simulink model "GTA_PCMFirmware"  (Simulink 7.8)
settings: Solver=FixedStepDiscrete  StartTime=0.0  StopTime=10.0  RelTol=1e-3
PreLoadFcn:
  | try, eval([bdroot '_setup']); catch, eval('model_setup', ''); end
InitFcn:
  | try, eval([bdroot '_setup']); catch, eval('model_setup', ''); end
undefined symbols (not defined in the file): fndFwd, fndNeut, fndRev, FWDlockout, GCM, keySwIgn2, motohawk_build_version, motohawk_trunc_name, motohawk_vardec_path, REVlockout
libraries: MotoHawk_lib x313, simulink x47, GTA_Library x13
(part 6 of 7)

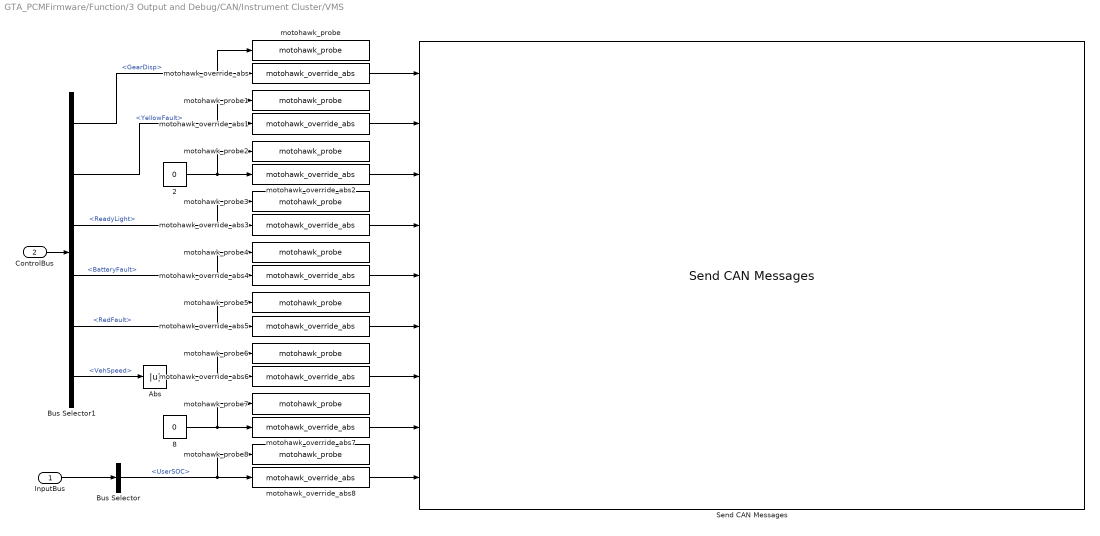
== system GTA_PCMFirmware/Function/3 Output and Debug/CAN/Instrument Cluster/VMS ==
  InputBus : Inport
  ControlBus : Inport  Port=2
  "   2" : Constant  Value=0  OutDataTypeStr=boolean
  "   8" : Constant  Value=0  OutDataTypeStr=uint8
  Abs : Abs
  Bus Selector : BusSelector  OutputSignals=CANin.BMS.csInfo.UserSOC
  Bus Selector1 : BusSelector  OutputSignals=Display.GearDisp,Display.FaultLamp.YellowFault,Display.ReadyLight,SYSin.BUS.Faults.BatteryFault.BatteryFault,Display.FaultLamp.RedFault,Display.VehSpeed
  Send CAN Messages : MotoHawk_lib/CAN Blocks/Send CAN Messages  bus=-2  nam='CAN_1'  msgl=CANMSG_ClusterVMS1  pace=5  labelwires=off
  motohawk_override_abs : MotoHawk_lib/Calibration & Probing Blocks/motohawk_override_abs  parent_name='GearboxDisplay'  parent_val=0  show_more=off  name_source=Use Parameter  parent_read_level=1  parent_override_level=1  view_as=Number  enum_struct={'Disabled', 'Enabled'}  use_help_units=off  parent_help=''  parent_units=''  use_min_max=off  parent_min=-inf  parent_max=inf  use_precision=off  parent_precision=''  parent_gain=1  parent_offset=0  parent_exp=1  use_mototune_group=off  parent_group=motohawk_vardec_path(gcb)
  motohawk_override_abs1 : MotoHawk_lib/Calibration & Probing Blocks/motohawk_override_abs  parent_name='YellowWarningLight'  parent_val=0  show_more=off  name_source=Use Parameter  parent_read_level=1  parent_override_level=1  view_as=Number  enum_struct={'Disabled', 'Enabled'}  use_help_units=off  parent_help=''  parent_units=''  use_min_max=off  parent_min=-inf  parent_max=inf  use_precision=off  parent_precision=''  parent_gain=1  parent_offset=0  parent_exp=1  use_mototune_group=off  parent_group=motohawk_vardec_path(gcb)
  motohawk_override_abs2 : MotoHawk_lib/Calibration & Probing Blocks/motohawk_override_abs  parent_name='SOCwarning'  parent_val=0  show_more=off  name_source=Use Parameter  parent_read_level=1  parent_override_level=1  view_as=Number  enum_struct={'Disabled', 'Enabled'}  use_help_units=off  parent_help=''  parent_units=''  use_min_max=off  parent_min=-inf  parent_max=inf  use_precision=off  parent_precision=''  parent_gain=1  parent_offset=0  parent_exp=1  use_mototune_group=off  parent_group=motohawk_vardec_path(gcb)
  motohawk_override_abs3 : MotoHawk_lib/Calibration & Probing Blocks/motohawk_override_abs  parent_name='ReadyLight'  parent_val=0  show_more=off  name_source=Use Parameter  parent_read_level=1  parent_override_level=1  view_as=Number  enum_struct={'Disabled', 'Enabled'}  use_help_units=off  parent_help=''  parent_units=''  use_min_max=off  parent_min=-inf  parent_max=inf  use_precision=off  parent_precision=''  parent_gain=1  parent_offset=0  parent_exp=1  use_mototune_group=off  parent_group=motohawk_vardec_path(gcb)
  motohawk_override_abs4 : MotoHawk_lib/Calibration & Probing Blocks/motohawk_override_abs  parent_name='BatteryWarning'  parent_val=0  show_more=off  name_source=Use Parameter  parent_read_level=1  parent_override_level=1  view_as=Number  enum_struct={'Disabled', 'Enabled'}  use_help_units=off  parent_help=''  parent_units=''  use_min_max=off  parent_min=-inf  parent_max=inf  use_precision=off  parent_precision=''  parent_gain=1  parent_offset=0  parent_exp=1  use_mototune_group=off  parent_group=motohawk_vardec_path(gcb)
  motohawk_override_abs5 : MotoHawk_lib/Calibration & Probing Blocks/motohawk_override_abs  parent_name='RedWarningLight'  parent_val=0  show_more=off  name_source=Use Parameter  parent_read_level=1  parent_override_level=1  view_as=Number  enum_struct={'Disabled', 'Enabled'}  use_help_units=off  parent_help=''  parent_units=''  use_min_max=off  parent_min=-inf  parent_max=inf  use_precision=off  parent_precision=''  parent_gain=1  parent_offset=0  parent_exp=1  use_mototune_group=off  parent_group=motohawk_vardec_path(gcb)
  motohawk_override_abs6 : MotoHawk_lib/Calibration & Probing Blocks/motohawk_override_abs  parent_name='VehicleSpeed'  parent_val=0  show_more=off  name_source=Use Parameter  parent_read_level=1  parent_override_level=1  view_as=Number  enum_struct={'Disabled', 'Enabled'}  use_help_units=off  parent_help=''  parent_units=''  use_min_max=off  parent_min=-inf  parent_max=inf  use_precision=off  parent_precision=''  parent_gain=1  parent_offset=0  parent_exp=1  use_mototune_group=off  parent_group=motohawk_vardec_path(gcb)
  motohawk_override_abs7 : MotoHawk_lib/Calibration & Probing Blocks/motohawk_override_abs  parent_name='Odometer'  parent_val=0  show_more=off  name_source=Use Parameter  parent_read_level=1  parent_override_level=1  view_as=Number  enum_struct={'Disabled', 'Enabled'}  use_help_units=off  parent_help=''  parent_units=''  use_min_max=off  parent_min=-inf  parent_max=inf  use_precision=off  parent_precision=''  parent_gain=1  parent_offset=0  parent_exp=1  use_mototune_group=off  parent_group=motohawk_vardec_path(gcb)
  motohawk_override_abs8 : MotoHawk_lib/Calibration & Probing Blocks/motohawk_override_abs  parent_name='SOC'  parent_val=0  show_more=off  name_source=Use Parameter  parent_read_level=1  parent_override_level=1  view_as=Number  enum_struct={'Disabled', 'Enabled'}  use_help_units=off  parent_help=''  parent_units=''  use_min_max=off  parent_min=-inf  parent_max=inf  use_precision=off  parent_precision=''  parent_gain=1  parent_offset=0  parent_exp=1  use_mototune_group=off  parent_group=motohawk_vardec_path(gcb)
  motohawk_probe : MotoHawk_lib/Calibration & Probing Blocks/motohawk_probe  nam='GearboxDisplay'  show_more=off  name_source=Use Parameter  read_level=1  view_as=Number  enum_struct={'Disabled', 'Enabled'}  vector_style=Wide Row  use_help_units=off  help=''  units=''  use_header_enum=off  row_header_enum={}  col_header_enum={}  use_min_max=off  min_val=-inf  max_val=inf  use_precision=off  precision=''  gain=1  offset=0  exp=1  use_mototune_group=off  mototune_group=motohawk_vardec_path(gcb)
  motohawk_probe1 : MotoHawk_lib/Calibration & Probing Blocks/motohawk_probe  nam='YellowWarningLight'  show_more=off  name_source=Use Parameter  read_level=1  view_as=Number  enum_struct={'Disabled', 'Enabled'}  vector_style=Wide Row  use_help_units=off  help=''  units=''  use_header_enum=off  row_header_enum={}  col_header_enum={}  use_min_max=off  min_val=-inf  max_val=inf  use_precision=off  precision=''  gain=1  offset=0  exp=1  use_mototune_group=off  mototune_group=motohawk_vardec_path(gcb)
  motohawk_probe2 : MotoHawk_lib/Calibration & Probing Blocks/motohawk_probe  nam='SOCwarning'  show_more=off  name_source=Use Parameter  read_level=1  view_as=Number  enum_struct={'Disabled', 'Enabled'}  vector_style=Wide Row  use_help_units=off  help=''  units=''  use_header_enum=off  row_header_enum={}  col_header_enum={}  use_min_max=off  min_val=-inf  max_val=inf  use_precision=off  precision=''  gain=1  offset=0  exp=1  use_mototune_group=off  mototune_group=motohawk_vardec_path(gcb)
  motohawk_probe3 : MotoHawk_lib/Calibration & Probing Blocks/motohawk_probe  nam='ReadyLight'  show_more=off  name_source=Use Parameter  read_level=1  view_as=Number  enum_struct={'Disabled', 'Enabled'}  vector_style=Wide Row  use_help_units=off  help=''  units=''  use_header_enum=off  row_header_enum={}  col_header_enum={}  use_min_max=off  min_val=-inf  max_val=inf  use_precision=off  precision=''  gain=1  offset=0  exp=1  use_mototune_group=off  mototune_group=motohawk_vardec_path(gcb)
  motohawk_probe4 : MotoHawk_lib/Calibration & Probing Blocks/motohawk_probe  nam='BatteryWarning'  show_more=off  name_source=Use Parameter  read_level=1  view_as=Number  enum_struct={'Disabled', 'Enabled'}  vector_style=Wide Row  use_help_units=off  help=''  units=''  use_header_enum=off  row_header_enum={}  col_header_enum={}  use_min_max=off  min_val=-inf  max_val=inf  use_precision=off  precision=''  gain=1  offset=0  exp=1  use_mototune_group=off  mototune_group=motohawk_vardec_path(gcb)
  motohawk_probe5 : MotoHawk_lib/Calibration & Probing Blocks/motohawk_probe  nam='RedWarningLight'  show_more=off  name_source=Use Parameter  read_level=1  view_as=Number  enum_struct={'Disabled', 'Enabled'}  vector_style=Wide Row  use_help_units=off  help=''  units=''  use_header_enum=off  row_header_enum={}  col_header_enum={}  use_min_max=off  min_val=-inf  max_val=inf  use_precision=off  precision=''  gain=1  offset=0  exp=1  use_mototune_group=off  mototune_group=motohawk_vardec_path(gcb)
  motohawk_probe6 : MotoHawk_lib/Calibration & Probing Blocks/motohawk_probe  nam='VehicleSpeed'  show_more=off  name_source=Use Parameter  read_level=1  view_as=Number  enum_struct={'Disabled', 'Enabled'}  vector_style=Wide Row  use_help_units=off  help=''  units=''  use_header_enum=off  row_header_enum={}  col_header_enum={}  use_min_max=off  min_val=-inf  max_val=inf  use_precision=off  precision=''  gain=1  offset=0  exp=1  use_mototune_group=off  mototune_group=motohawk_vardec_path(gcb)
  motohawk_probe7 : MotoHawk_lib/Calibration & Probing Blocks/motohawk_probe  nam='Odometer'  show_more=off  name_source=Use Parameter  read_level=1  view_as=Number  enum_struct={'Disabled', 'Enabled'}  vector_style=Wide Row  use_help_units=off  help=''  units=''  use_header_enum=off  row_header_enum={}  col_header_enum={}  use_min_max=off  min_val=-inf  max_val=inf  use_precision=off  precision=''  gain=1  offset=0  exp=1  use_mototune_group=off  mototune_group=motohawk_vardec_path(gcb)
  motohawk_probe8 : MotoHawk_lib/Calibration & Probing Blocks/motohawk_probe  nam='SOC'  show_more=off  name_source=Use Parameter  read_level=1  view_as=Number  enum_struct={'Disabled', 'Enabled'}  vector_style=Wide Row  use_help_units=off  help=''  units=''  use_header_enum=off  row_header_enum={}  col_header_enum={}  use_min_max=off  min_val=-inf  max_val=inf  use_precision=off  precision=''  gain=1  offset=0  exp=1  use_mototune_group=off  mototune_group=motohawk_vardec_path(gcb)
  wires:
  InputBus/1 -> Bus Selector/1
  motohawk_override_abs/1 -> Send CAN Messages/1
  motohawk_override_abs1/1 -> Send CAN Messages/2
  motohawk_override_abs2/1 -> Send CAN Messages/3
  motohawk_override_abs3/1 -> Send CAN Messages/4
  motohawk_override_abs4/1 -> Send CAN Messages/5
  motohawk_override_abs5/1 -> Send CAN Messages/6
  motohawk_override_abs6/1 -> Send CAN Messages/7
  motohawk_override_abs7/1 -> Send CAN Messages/8
  motohawk_override_abs8/1 -> Send CAN Messages/9
  Bus Selector/1 -> motohawk_override_abs8/1, motohawk_probe8/1  "<UserSOC>"
  Bus Selector1/2 -> motohawk_override_abs1/1, motohawk_probe1/1  "<YellowFault>"
  "   8"/1 -> motohawk_override_abs7/1, motohawk_probe7/1
  Bus Selector1/6 -> Abs/1  "<VehSpeed>"
  Bus Selector1/5 -> motohawk_override_abs5/1, motohawk_probe5/1  "<RedFault>"
  Bus Selector1/4 -> motohawk_override_abs4/1, motohawk_probe4/1  "<BatteryFault>"
  Bus Selector1/3 -> motohawk_override_abs3/1, motohawk_probe3/1  "<ReadyLight>"
  "   2"/1 -> motohawk_override_abs2/1, motohawk_probe2/1
  ControlBus/1 -> Bus Selector1/1
  Bus Selector1/1 -> motohawk_override_abs/1, motohawk_probe/1  "<GearDisp>"
  Abs/1 -> motohawk_override_abs6/1, motohawk_probe6/1

== system GTA_PCMFirmware/Function/3 Output and Debug/CAN/MotorController/Controller Command ==
  In1 : Inport
  Bus Selector : BusSelector  OutputSignals=MotorControl.enable,MotorControl.fndOutput,MotorControl.torqueRequest,SYSin.BUS.Input Bus.Limits.BattLimits.MaxRegenVoltage,SYSin.BUS.Input Bus.SysParams.maxMotorRPM
  Send CAN Messages : MotoHawk_lib/CAN Blocks/Send CAN Messages  bus=-2  nam='Isolated_CAN'  msgl=CANMSG_TrqCmd  pace=10  labelwires=off
  motohawk_override_abs : MotoHawk_lib/Calibration & Probing Blocks/motohawk_override_abs  parent_name='mcEnable'  parent_val=0  show_more=off  name_source=Use Parameter  parent_read_level=1  parent_override_level=1  view_as=Number  enum_struct={'Disabled', 'Enabled'}  use_help_units=off  parent_help=''  parent_units=''  use_min_max=off  parent_min=-inf  parent_max=inf  use_precision=off  parent_precision=''  parent_gain=1  parent_offset=0  parent_exp=1  use_mototune_group=off  parent_group=motohawk_vardec_path(gcb)
  motohawk_override_abs1 : MotoHawk_lib/Calibration & Probing Blocks/motohawk_override_abs  parent_name='mcGearBoxPos'  parent_val=0  show_more=off  name_source=Use Parameter  parent_read_level=1  parent_override_level=1  view_as=Number  enum_struct={'Disabled', 'Enabled'}  use_help_units=off  parent_help=''  parent_units=''  use_min_max=off  parent_min=-inf  parent_max=inf  use_precision=off  parent_precision=''  parent_gain=1  parent_offset=0  parent_exp=1  use_mototune_group=off  parent_group=motohawk_vardec_path(gcb)
  motohawk_override_abs2 : MotoHawk_lib/Calibration & Probing Blocks/motohawk_override_abs  parent_name='mcCurrentCommand'  parent_val=0  show_more=off  name_source=Use Parameter  parent_read_level=1  parent_override_level=1  view_as=Number  enum_struct={'Disabled', 'Enabled'}  use_help_units=off  parent_help=''  parent_units=''  use_min_max=off  parent_min=-inf  parent_max=inf  use_precision=off  parent_precision=''  parent_gain=1  parent_offset=0  parent_exp=1  use_mototune_group=off  parent_group=motohawk_vardec_path(gcb)
  motohawk_override_abs3 : MotoHawk_lib/Calibration & Probing Blocks/motohawk_override_abs  parent_name='mcMaxRegenVolts'  parent_val=0  show_more=off  name_source=Use Parameter  parent_read_level=1  parent_override_level=1  view_as=Number  enum_struct={'Disabled', 'Enabled'}  use_help_units=off  parent_help=''  parent_units=''  use_min_max=off  parent_min=-inf  parent_max=inf  use_precision=off  parent_precision=''  parent_gain=1  parent_offset=0  parent_exp=1  use_mototune_group=off  parent_group=motohawk_vardec_path(gcb)
  motohawk_override_abs4 : MotoHawk_lib/Calibration & Probing Blocks/motohawk_override_abs  parent_name='mcMaxSpeed'  parent_val=0  show_more=off  name_source=Use Parameter  parent_read_level=1  parent_override_level=1  view_as=Number  enum_struct={'Disabled', 'Enabled'}  use_help_units=off  parent_help=''  parent_units=''  use_min_max=off  parent_min=-inf  parent_max=inf  use_precision=off  parent_precision=''  parent_gain=1  parent_offset=0  parent_exp=1  use_mototune_group=off  parent_group=motohawk_vardec_path(gcb)
  motohawk_probe : MotoHawk_lib/Calibration & Probing Blocks/motohawk_probe  nam='mcEnable'  show_more=off  name_source=Use Parameter  read_level=1  view_as=Number  enum_struct={'Disabled', 'Enabled'}  vector_style=Wide Row  use_help_units=off  help=''  units=''  use_header_enum=off  row_header_enum={}  col_header_enum={}  use_min_max=off  min_val=-inf  max_val=inf  use_precision=off  precision=''  gain=1  offset=0  exp=1  use_mototune_group=off  mototune_group=motohawk_vardec_path(gcb)
  motohawk_probe1 : MotoHawk_lib/Calibration & Probing Blocks/motohawk_probe  nam='mcGearBoxPos'  show_more=off  name_source=Use Parameter  read_level=1  view_as=Number  enum_struct={'Disabled', 'Enabled'}  vector_style=Wide Row  use_help_units=off  help=''  units=''  use_header_enum=off  row_header_enum={}  col_header_enum={}  use_min_max=off  min_val=-inf  max_val=inf  use_precision=off  precision=''  gain=1  offset=0  exp=1  use_mototune_group=off  mototune_group=motohawk_vardec_path(gcb)
  motohawk_probe2 : MotoHawk_lib/Calibration & Probing Blocks/motohawk_probe  nam='mcCurrentCommand'  show_more=off  name_source=Use Parameter  read_level=1  view_as=Number  enum_struct={'Disabled', 'Enabled'}  vector_style=Wide Row  use_help_units=off  help=''  units=''  use_header_enum=off  row_header_enum={}  col_header_enum={}  use_min_max=off  min_val=-inf  max_val=inf  use_precision=off  precision=''  gain=1  offset=0  exp=1  use_mototune_group=off  mototune_group=motohawk_vardec_path(gcb)
  motohawk_probe3 : MotoHawk_lib/Calibration & Probing Blocks/motohawk_probe  nam='mcMaxRegenVolts'  show_more=off  name_source=Use Parameter  read_level=1  view_as=Number  enum_struct={'Disabled', 'Enabled'}  vector_style=Wide Row  use_help_units=off  help=''  units=''  use_header_enum=off  row_header_enum={}  col_header_enum={}  use_min_max=off  min_val=-inf  max_val=inf  use_precision=off  precision=''  gain=1  offset=0  exp=1  use_mototune_group=off  mototune_group=motohawk_vardec_path(gcb)
  motohawk_probe4 : MotoHawk_lib/Calibration & Probing Blocks/motohawk_probe  nam='mcMaxSpeed'  show_more=off  name_source=Use Parameter  read_level=1  view_as=Number  enum_struct={'Disabled', 'Enabled'}  vector_style=Wide Row  use_help_units=off  help=''  units=''  use_header_enum=off  row_header_enum={}  col_header_enum={}  use_min_max=off  min_val=-inf  max_val=inf  use_precision=off  precision=''  gain=1  offset=0  exp=1  use_mototune_group=off  mototune_group=motohawk_vardec_path(gcb)
  wires:
  In1/1 -> Bus Selector/1
  motohawk_override_abs/1 -> Send CAN Messages/1
  motohawk_override_abs1/1 -> Send CAN Messages/2
  motohawk_override_abs2/1 -> Send CAN Messages/3
  motohawk_override_abs3/1 -> Send CAN Messages/4
  motohawk_override_abs4/1 -> Send CAN Messages/5
  Bus Selector/5 -> motohawk_override_abs4/1, motohawk_probe4/1  "<maxMotorRPM>"
  Bus Selector/1 -> motohawk_override_abs/1, motohawk_probe/1  "<enable>"
  Bus Selector/2 -> motohawk_override_abs1/1, motohawk_probe1/1  "<fndOutput>"
  Bus Selector/3 -> motohawk_override_abs2/1, motohawk_probe2/1  "<torqueRequest>"
  Bus Selector/4 -> motohawk_override_abs3/1, motohawk_probe3/1  "<MaxRegenVoltage>"

== system GTA_PCMFirmware/Function/3 Output and Debug/CAN/MotorController/Watchdog ==
  In1 : Inport
  Bus Selector : BusSelector  OutputSignals=CANin.Motor Controller.KinWatchdog.WDcounter
  Send CAN Messages : MotoHawk_lib/CAN Blocks/Send CAN Messages  bus=-2  nam='Isolated_CAN'  msgl=CANMSG_Watchdog_ACK  pace=10  labelwires=off
  motohawk_probe : MotoHawk_lib/Calibration & Probing Blocks/motohawk_probe  nam='MCwatchdogOut'  show_more=off  name_source=Use Parameter  read_level=1  view_as=Number  enum_struct={'Disabled', 'Enabled'}  vector_style=Wide Row  use_help_units=off  help=''  units=''  use_header_enum=off  row_header_enum={}  col_header_enum={}  use_min_max=off  min_val=-inf  max_val=inf  use_precision=off  precision=''  gain=1  offset=0  exp=1  use_mototune_group=off  mototune_group=motohawk_vardec_path(gcb)
  wires:
  In1/1 -> Bus Selector/1
  Bus Selector/1 -> Send CAN Messages/1, motohawk_probe/1  "<WDcounter>"

== system GTA_PCMFirmware/Function/1 Inputs and Paramaters/CAN/ Motor Controller/VoltageSpeedFB/SpeedLPF ==
  Speed : Inport
  Add : Sum  Inputs=+
  Gain : Gain  Gain=1/100
  Tapped Delay : simulink/Discrete/Tapped Delay  vinit=0.0  samptime=-1  NumDelays=100  DelayOrder=Oldest  includeCurrent=off
  SpeedLPF : Outport
  wires:
  Tapped Delay/1 -> Add/1
  Add/1 -> Gain/1
  Speed/1 -> Tapped Delay/1
  Gain/1 -> SpeedLPF/1

== system GTA_PCMFirmware/Function/1 Inputs and Paramaters/CAN/BMS/  Current Sensor/UserSOC ==
  csSOC : Inport
  MinSOC : Inport  Port=2
  Constant : Constant  Value=0  OutDataTypeStr=single
  Constant1 : Constant  Value=100  OutDataTypeStr=single
  Constant2 : Constant  Value=[0 0 100]  OutDataTypeStr=single
  Lookup Table Dynamic : simulink/Lookup Tables/Lookup Table Dynamic  LookUpMeth=Interpolation-Use End Values  OutDataTypeStr=fixdt('single')  OutputDataTypeScalingMode=Specify via dialog  OutDataType=fixdt('single')  OutScaling=[]  DoSatur=off
  Mux : Mux  Inputs=3
  UserSOC : Outport
  wires:
  Constant/1 -> Mux/1
  Constant1/1 -> Mux/3
  Mux/1 -> Lookup Table Dynamic/2
  Constant2/1 -> Lookup Table Dynamic/3
  csSOC/1 -> Lookup Table Dynamic/1
  Lookup Table Dynamic/1 -> UserSOC/1  "UserSOC"
  MinSOC/1 -> Mux/2

== system GTA_PCMFirmware/Function/2 Control Loop/Component Controls/Display Control/Fault Lamps/BMS Error ==
  In1 : Inport
  Bus Selector1 : BusSelector  OutputSignals=BUS.Input Bus.CANin.BMS.csChargeFlags.CellHigh
  Constant : Constant  Value=0  OutDataTypeStr=boolean
  Terminator : Terminator
  Out1 : Outport
  wires:
  Bus Selector1/1 -> Terminator/1  "<CellHigh>"
  In1/1 -> Bus Selector1/1
  Constant/1 -> Out1/1

== system GTA_PCMFirmware/Function/2 Control Loop/Component Controls/Display Control/Fault Lamps/BMSFault ==
  In1 : Inport
  Bus Selector1 : BusSelector  OutputSignals=BUS.Input Bus.CANin.BMS.csInfo.csCANok
  Logical Operator : Logic  Operator=NOT  AllPortsSameDT=off  OutDataTypeStr=boolean
  Out1 : Outport
  wires:
  Bus Selector1/1 -> Logical Operator/1  "<csCANok>"
  In1/1 -> Bus Selector1/1
  Logical Operator/1 -> Out1/1

== system GTA_PCMFirmware/Function/2 Control Loop/Component Controls/Display Control/Fault Lamps/E-Stop ==
  In1 : Inport
  Bus Selector1 : BusSelector  OutputSignals=BUS.Input Bus.DigitalIn.EStop.EStop
  Out1 : Outport
  wires:
  Bus Selector1/1 -> Out1/1  "<EStop>"
  In1/1 -> Bus Selector1/1

== system GTA_PCMFirmware/Function/2 Control Loop/Component Controls/Display Control/Fault Lamps/KinetekCodeEnable ==
  In1 : Inport
  Bus Selector1 : BusSelector  OutputSignals=ModeControl.StatusBits.DriveMode
  Delay : Delay  DelayLength=1000
  Logical Operator : Logic  AllPortsSameDT=off  OutDataTypeStr=boolean
  Out1 : Outport
  wires:
  In1/1 -> Bus Selector1/1
  Delay/1 -> Logical Operator/2
  Bus Selector1/1 -> Delay/1, Logical Operator/1  "<DriveMode>"
  Logical Operator/1 -> Out1/1

== system GTA_PCMFirmware/Function/2 Control Loop/Component Controls/Display Control/Fault Lamps/KinetekError ==
  In1 : Inport
  Bus Selector1 : BusSelector  OutputSignals=BUS.Input Bus.CANin.Motor Controller.KinTempWarn.WarningFlags
  Constant : Constant  Value=0  OutDataTypeStr=boolean
  Logical Operator : Logic  Operator=OR  Inputs=1  AllPortsSameDT=off  OutDataTypeStr=boolean
  Logical Operator1 : Logic  Operator=OR  Inputs=3  AllPortsSameDT=off  OutDataTypeStr=boolean
  Out1 : Outport
  wires:
  Logical Operator/1 -> Logical Operator1/3
  In1/1 -> Bus Selector1/1
  Logical Operator1/1 -> Out1/1
  Bus Selector1/1 -> Logical Operator/1  "<WarningFlags>"
  Constant/1 -> Logical Operator1/1, Logical Operator1/2

== system GTA_PCMFirmware/Function/2 Control Loop/Component Controls/Display Control/Fault Lamps/KinetekFault ==
  In1 : Inport
  Bus Selector1 : BusSelector  OutputSignals=BUS.Input Bus.CANin.Motor Controller.KinWatchdog.WatchdogCANok,BUS.Input Bus.CANin.Motor Controller.KinVoltSpeed.ErrorField
  Data Type Conversion : DataTypeConversion  OutDataTypeStr=uint16
  Logical Operator : Logic  Operator=OR  Inputs=1  AllPortsSameDT=off  OutDataTypeStr=boolean
  Logical Operator1 : Logic  Operator=OR  AllPortsSameDT=off  OutDataTypeStr=boolean
  Logical Operator2 : Logic  Operator=NOT  Inputs=1  AllPortsSameDT=off  OutDataTypeStr=boolean
  Out1 : Outport
  wires:
  Bus Selector1/2 -> Data Type Conversion/1  "<ErrorField>"
  Bus Selector1/1 -> Logical Operator2/1  "<WatchdogCANok>"
  Logical Operator/1 -> Logical Operator1/2
  In1/1 -> Bus Selector1/1
  Logical Operator1/1 -> Out1/1
  Logical Operator2/1 -> Logical Operator1/1
  Data Type Conversion/1 -> Logical Operator/1

== system GTA_PCMFirmware/Function/2 Control Loop/Component Controls/Display Control/Fault Lamps/PCMError ==
  note: VoltFault
  In1 : Inport
  Bus Selector1 : BusSelector  OutputSignals=BUS.Input Bus.AnalogIn.ThrottlePedal.dbgAPPok,BUS.Input Bus.DigitalIn.EStop.EStop,BUS.Input Bus.DigitalIn.Shifter.dbgShifter.sbgShiftErr,BUS.Voltage level.VoltageFault,ModeControl.StatusBits.DriveMode
  Delay : Delay  DelayLength=1000
  Logical Operator : Logic  AllPortsSameDT=off  OutDataTypeStr=boolean
  Logical Operator1 : Logic  Operator=OR  Inputs=4  AllPortsSameDT=off  OutDataTypeStr=boolean
  Logical Operator2 : Logic  Operator=NOT  Inputs=1  AllPortsSameDT=off  OutDataTypeStr=boolean
  Logical Operator3 : Logic  AllPortsSameDT=off  OutDataTypeStr=boolean
  Out1 : Outport
  wires:
  In1/1 -> Bus Selector1/1
  Logical Operator1/1 -> Out1/1
  Bus Selector1/1 -> Logical Operator2/1  "<dbgAPPok>"
  Bus Selector1/2 -> Logical Operator1/2  "<EStop>"
  Logical Operator2/1 -> Logical Operator1/1
  Delay/1 -> Logical Operator/2
  Logical Operator/1 -> Logical Operator1/3
  Bus Selector1/3 -> Delay/1, Logical Operator/1  "<sbgShiftErr>"
  Bus Selector1/4 -> Logical Operator3/1  "<VoltageFault>"
  Bus Selector1/5 -> Logical Operator3/2  "<DriveMode>"
  Logical Operator3/1 -> Logical Operator1/4

== system GTA_PCMFirmware/Function/2 Control Loop/Component Controls/Display Control/Fault Lamps/PCMFault ==
  In1 : Inport
  Bus Selector1 : BusSelector  OutputSignals=ModeControl.StatusBits.BatteryFault,ModeControl.StatusBits.ContactorFault
  Logical Operator : Logic  Operator=OR  Inputs=1  AllPortsSameDT=off  OutDataTypeStr=boolean
  Mux : Mux  Inputs=2
  Out1 : Outport
  wires:
  In1/1 -> Bus Selector1/1
  Bus Selector1/1 -> Mux/1  "<BatteryFault>"
  Bus Selector1/2 -> Mux/2  "<ContactorFault>"
  Mux/1 -> Logical Operator/1
  Logical Operator/1 -> Out1/1

== system GTA_PCMFirmware/Function/2 Control Loop/Component Controls/Motor Control/Current Request Algorithm/Throttle Pedal Mapping ==
  FNDOut : Inport
  Pedal Percent : Inport  Port=2
  Speed : Inport  Port=3
  Product1 : Product  OutDataTypeStr=single  RndMeth=Zero
  Relay : Relay  OnSwitchValue=2  OffSwitchValue=1  OffOutputValue=-1  OutDataTypeStr=single
  motohawk_interpolation_2d1 : MotoHawk_lib/Lookup Tables/motohawk_interpolation_2d  nam='ForwardThrottle'  table_data=[30 30 30 47.4 65 82.6 100; 0 0 12 34 56 78 100; -10 0 6 29.4 53 76.4 100; -30 -19 -8 25 50 75 100; -60 -49 -38 20 46.6 73.4 100; -100 -89 -78 12 41.4 70.6 100]  show_more=on  data_type=double  storage=NonAdaptive  read_level=1  write_level=1  ovr_cals=on  use_help=off  help=''  units=''  use_min_max=off  min_val=-inf  max_val=inf  use_precision=off  precision=''  gain=1  offset=0  exp=1  use_links=off  row_prelookup_block=''  col_prelookup_block=''  output_name=''  use_mototune_group=off  mototune_group=motohawk_vardec_path(gcb)
  motohawk_prelookup2 : MotoHawk_lib/Lookup Tables/motohawk_prelookup  nam='SpeedFwdPrelookup'  breakpoint_data=[-100 0 100 200 1000 5000]  show_more=on  data_type=single  storage=Constant  read_level=1  write_level=1  ovr_cals=on  use_help=off  help=''  units=''  use_min_max=off  min_val=-inf  max_val=inf  use_precision=off  precision=''  gain=1  offset=0  exp=1  use_links=off  input_name=''  use_mototune_group=off  mototune_group=motohawk_vardec_path(gcb)
  motohawk_prelookup3 : MotoHawk_lib/Lookup Tables/motohawk_prelookup  nam='PedalPositionFwdPrelookup'  breakpoint_data=[0 2 5 10 20 80 100]  show_more=on  data_type=single  storage=Constant  read_level=1  write_level=1  ovr_cals=on  use_help=off  help=''  units=''  use_min_max=off  min_val=-inf  max_val=inf  use_precision=off  precision=''  gain=1  offset=0  exp=1  use_links=off  input_name=''  use_mototune_group=off  mototune_group=motohawk_vardec_path(gcb)
  motohawk_probe1 : MotoHawk_lib/Calibration & Probing Blocks/motohawk_probe  nam='TorqueLookupInput'  show_more=on  name_source=Use Parameter  read_level=1  view_as=Number  enum_struct={'Disabled', 'Enabled'}  vector_style=Wide Row  use_help_units=off  help=''  units=''  use_header_enum=off  row_header_enum={}  col_header_enum={}  use_min_max=off  min_val=-inf  max_val=inf  use_precision=off  precision=''  gain=1  offset=0  exp=1  use_mototune_group=off  mototune_group=motohawk_vardec_path(gcb)
  motohawk_probe2 : MotoHawk_lib/Calibration & Probing Blocks/motohawk_probe  nam='throttle_lookup_out'  show_more=on  name_source=Use Parameter  read_level=1  view_as=Number  enum_struct={'Disabled', 'Enabled'}  vector_style=Wide Row  use_help_units=off  help=''  units=''  use_header_enum=off  row_header_enum={}  col_header_enum={}  use_min_max=off  min_val=-inf  max_val=inf  use_precision=off  precision=''  gain=1  offset=0  exp=1  use_mototune_group=off  mototune_group=motohawk_vardec_path(gcb)
  Out1 : Outport
  wires:
  Relay/1 -> Product1/1
  Product1/1 -> motohawk_prelookup2/1
  FNDOut/1 -> Relay/1
  Speed/1 -> Product1/2
  motohawk_interpolation_2d1/1 -> Out1/1, motohawk_probe2/1
  Pedal Percent/1 -> motohawk_probe1/1, motohawk_prelookup3/1
  motohawk_prelookup2/1 -> motohawk_interpolation_2d1/1
  motohawk_prelookup3/1 -> motohawk_interpolation_2d1/2

== system GTA_PCMFirmware/Function/2 Control Loop/Safety/Current Limit/RegenLimit/Cell Voltage limiter ==
  InputBus : Inport
  Bus Selector : BusSelector  OutputSignals=Input Bus.CANin.BMS.csCellInfo.HighCellValue,Input Bus.SysParams.CellVoltageTaper,Input Bus.SysParams.CellVoltDB,Input Bus.Limits.BattLimits.MaxCellVoltage
  Constant : Constant  Value=[100 0]  OutDataTypeStr=single
  Lookup Table Dynamic : simulink/Lookup Tables/Lookup Table Dynamic  LookUpMeth=Interpolation-Use End Values  OutDataTypeStr=fixdt('single')  OutputDataTypeScalingMode=Specify via dialog  OutDataType=fixdt('single')  OutScaling=[]  DoSatur=off
  Mux : Mux  Inputs=2
  Sum : Sum  Inputs=|-+
  Sum1 : Sum  Inputs=-+|
  PercOut : Outport
  wires:
  InputBus/1 -> Bus Selector/1
  Sum/1 -> Mux/1
  Sum1/1 -> Mux/2, Sum/2
  Mux/1 -> Lookup Table Dynamic/2
  Constant/1 -> Lookup Table Dynamic/3
  Bus Selector/1 -> Lookup Table Dynamic/1  "<HighCellValue>"
  Lookup Table Dynamic/1 -> PercOut/1
  Bus Selector/4 -> Sum1/2  "<MaxCellVoltage>"
  Bus Selector/3 -> Sum1/1  "<CellVoltDB>"
  Bus Selector/2 -> Sum/1  "<CellVoltageTaper>"

== system GTA_PCMFirmware/Function/2 Control Loop/Safety/Current Limit/RegenLimit/Current Limiter ==
  InputBus : Inport
  Bus Selector1 : BusSelector  OutputSignals=Input Bus.CANin.BMS.csInfo.csCurrent,Input Bus.SysParams.PackCurrentTaper,Input Bus.Limits.BattLimits.RegenLimit
  Constant : Constant  Value=[100 0]  OutDataTypeStr=single
  Lookup Table Dynamic : simulink/Lookup Tables/Lookup Table Dynamic  LookUpMeth=Interpolation-Use End Values  OutDataTypeStr=fixdt('single')  OutputDataTypeScalingMode=Specify via dialog  OutDataType=fixdt('single')  OutScaling=[]  DoSatur=off
  Mux : Mux  Inputs=2
  Sum : Sum  Inputs=|-+
  PercOut : Outport
  wires:
  InputBus/1 -> Bus Selector1/1
  Bus Selector1/1 -> Lookup Table Dynamic/1  "<csCurrent>"
  Mux/1 -> Lookup Table Dynamic/2
  Constant/1 -> Lookup Table Dynamic/3
  Lookup Table Dynamic/1 -> PercOut/1
  Bus Selector1/3 -> Mux/2, Sum/2  "<RegenLimit>"
  Bus Selector1/2 -> Sum/1  "<PackCurrentTaper>"
  Sum/1 -> Mux/1

== system GTA_PCMFirmware/Function/2 Control Loop/Safety/Current Limit/RegenLimit/High Cell Temp ==
  InputBus : Inport
  Bus Selector : BusSelector  OutputSignals=Input Bus.CANin.BMS.csCellTemps.HighCellTemp,Input Bus.SysParams.CellTempTaper,Input Bus.Limits.BattLimits.MaxChargeTemp
  Constant : Constant  Value=[100 0]  OutDataTypeStr=single
  Lookup Table Dynamic : simulink/Lookup Tables/Lookup Table Dynamic  LookUpMeth=Interpolation-Use End Values  OutDataTypeStr=fixdt('single')  OutputDataTypeScalingMode=Specify via dialog  OutDataType=fixdt('single')  OutScaling=[]  DoSatur=off
  Mux : Mux  Inputs=2
  Sum : Sum  Inputs=|-+
  PercOut : Outport
  wires:
  InputBus/1 -> Bus Selector/1
  Bus Selector/3 -> Mux/2, Sum/2  "<MaxChargeTemp>"
  Sum/1 -> Mux/1
  Bus Selector/2 -> Sum/1  "<CellTempTaper>"
  Constant/1 -> Lookup Table Dynamic/3
  Mux/1 -> Lookup Table Dynamic/2
  Bus Selector/1 -> Lookup Table Dynamic/1  "<HighCellTemp>"
  Lookup Table Dynamic/1 -> PercOut/1

== system GTA_PCMFirmware/Function/2 Control Loop/Safety/Current Limit/RegenLimit/Low Cell Temp ==
  InputBus : Inport
  Bus Selector1 : BusSelector  OutputSignals=Input Bus.CANin.BMS.csCellTemps.LowCellTemp,Input Bus.Limits.BattLimits.MinChargeTemp,Input Bus.SysParams.CellTempTaper
  Constant : Constant  Value=[0 100]  OutDataTypeStr=single
  Lookup Table Dynamic : simulink/Lookup Tables/Lookup Table Dynamic  LookUpMeth=Interpolation-Use End Values  OutDataTypeStr=fixdt('single')  OutputDataTypeScalingMode=Specify via dialog  OutDataType=fixdt('single')  OutScaling=[]  DoSatur=off
  Mux : Mux  Inputs=2
  Sum : Sum  Inputs=++|
  PercOut : Outport
  wires:
  InputBus/1 -> Bus Selector1/1
  Constant/1 -> Lookup Table Dynamic/3
  Mux/1 -> Lookup Table Dynamic/2
  Bus Selector1/1 -> Lookup Table Dynamic/1  "<LowCellTemp>"
  Bus Selector1/2 -> Mux/1, Sum/1  "<MinChargeTemp>"
  Sum/1 -> Mux/2
  Bus Selector1/3 -> Sum/2  "<CellTempTaper>"
  Lookup Table Dynamic/1 -> PercOut/1

== system GTA_PCMFirmware/Function/2 Control Loop/Safety/Current Limit/RegenLimit/Pack Voltage Limiter ==
  InputBus : Inport
  Bus Selector : BusSelector  OutputSignals=Voltage level.AvgVoltage,Input Bus.SysParams.PackVoltageTaper,Input Bus.Limits.BattLimits.MaxPackVoltage
  Constant : Constant  Value=[100 0]  OutDataTypeStr=single
  Lookup Table Dynamic : simulink/Lookup Tables/Lookup Table Dynamic  LookUpMeth=Interpolation-Use End Values  OutDataTypeStr=fixdt('single')  OutputDataTypeScalingMode=Specify via dialog  OutDataType=fixdt('single')  OutScaling=[]  DoSatur=off
  Mux : Mux  Inputs=2
  Sum : Sum  Inputs=|-+
  PercOut : Outport
  wires:
  InputBus/1 -> Bus Selector/1
  Bus Selector/1 -> Lookup Table Dynamic/1  "<AvgVoltage>"
  Mux/1 -> Lookup Table Dynamic/2
  Constant/1 -> Lookup Table Dynamic/3
  Lookup Table Dynamic/1 -> PercOut/1
  Bus Selector/3 -> Mux/2, Sum/2  "<MaxPackVoltage>"
  Bus Selector/2 -> Sum/1  "<PackVoltageTaper>"
  Sum/1 -> Mux/1

== system GTA_PCMFirmware/Function/2 Control Loop/Safety/Current Limit/RegenLimit/SOC Limiter ==
  InputBus : Inport
  Bus Selector : BusSelector  OutputSignals=Input Bus.CANin.BMS.csInfo.csSOC
  motohawk_table_1d : MotoHawk_lib/Lookup Tables/motohawk_table_1d  nam='HighSOCregenlimit'  bp_nam=''  breakpoint_data=[97 98 99]  table_data=[100 100 0]  show_more=on  bp_data_type=single  bp_storage=Constant  table_data_type=single  storage=NonAdaptive  read_level=1  write_level=1  ovr_cals=on  use_help=off  help=''  bp_units=''  table_units=''  use_min_max=off  bp_min_val=-inf  bp_max_val=inf  min_val=-inf  max_val=inf  use_precision=off  use_breakpoint=off  b_precision=''  b_gain=1  b_offset=0  b_exp=1  use_table=off  t_precision=''  t_gain=1  t_offset=0  t_exp=1  use_links=off  input_name=''  output_name=''  use_mototune_group=off  mototune_group=motohawk_vardec_path(gcb)
  PercOut : Outport
  wires:
  InputBus/1 -> Bus Selector/1
  motohawk_table_1d/1 -> PercOut/1
  Bus Selector/1 -> motohawk_table_1d/1  "<csSOC>"

== system GTA_PCMFirmware/Function/2 Control Loop/Safety/Current Limit/TorqueLimit/Cell Voltage limiter ==
  InputBus : Inport
  Bus Selector : BusSelector  OutputSignals=Input Bus.CANin.BMS.csCellInfo.LowCellValue,Input Bus.Limits.BattLimits.MinCellVoltage,Input Bus.SysParams.CellVoltDB,Input Bus.SysParams.CellVoltageTaper
  Constant : Constant  Value=[0 100]  OutDataTypeStr=single
  Lookup Table Dynamic : simulink/Lookup Tables/Lookup Table Dynamic  LookUpMeth=Interpolation-Use End Values  OutDataTypeStr=fixdt('single')  OutputDataTypeScalingMode=Specify via dialog  OutDataType=fixdt('single')  OutScaling=[]  DoSatur=off
  Mux : Mux  Inputs=2
  Sum : Sum  Inputs=|++
  Sum1 : Sum  Inputs=++|
  PercOut : Outport
  wires:
  InputBus/1 -> Bus Selector/1
  Bus Selector/2 -> Sum/1  "<MinCellVoltage>"
  Bus Selector/3 -> Sum/2  "<CellVoltDB>"
  Sum/1 -> Mux/1, Sum1/1
  Bus Selector/4 -> Sum1/2  "<CellVoltageTaper>"
  Sum1/1 -> Mux/2
  Mux/1 -> Lookup Table Dynamic/2
  Constant/1 -> Lookup Table Dynamic/3
  Bus Selector/1 -> Lookup Table Dynamic/1  "<LowCellValue>"
  Lookup Table Dynamic/1 -> PercOut/1

== system GTA_PCMFirmware/Function/2 Control Loop/Safety/Current Limit/TorqueLimit/Current Limiter ==
  InputBus : Inport
  Bus Selector1 : BusSelector  OutputSignals=Input Bus.CANin.BMS.csInfo.csCurrent,Input Bus.Limits.BattLimits.CurrentLimit,Input Bus.SysParams.PackCurrentTaper
  Constant : Constant  Value=[0 100]  OutDataTypeStr=single
  Lookup Table Dynamic : simulink/Lookup Tables/Lookup Table Dynamic  LookUpMeth=Interpolation-Use End Values  OutDataTypeStr=fixdt('single')  OutputDataTypeScalingMode=Specify via dialog  OutDataType=fixdt('single')  OutScaling=[]  DoSatur=off
  Mux : Mux  Inputs=2
  Sum : Sum  Inputs=++|
  PercOut : Outport
  wires:
  InputBus/1 -> Bus Selector1/1
  Bus Selector1/1 -> Lookup Table Dynamic/1  "<csCurrent>"
  Mux/1 -> Lookup Table Dynamic/2
  Constant/1 -> Lookup Table Dynamic/3
  Lookup Table Dynamic/1 -> PercOut/1
  Bus Selector1/2 -> Mux/1, Sum/1  "<CurrentLimit>"
  Bus Selector1/3 -> Sum/2  "<PackCurrentTaper>"
  Sum/1 -> Mux/2

== system GTA_PCMFirmware/Function/2 Control Loop/Safety/Current Limit/TorqueLimit/High Cell Temp ==
  InputBus : Inport
  Bus Selector : BusSelector  OutputSignals=Input Bus.CANin.BMS.csCellTemps.HighCellTemp,Input Bus.SysParams.CellTempTaper,Input Bus.Limits.BattLimits.MaxDischargeTemp
  Constant : Constant  Value=[100 0]  OutDataTypeStr=single
  Lookup Table Dynamic : simulink/Lookup Tables/Lookup Table Dynamic  LookUpMeth=Interpolation-Use End Values  OutDataTypeStr=fixdt('single')  OutputDataTypeScalingMode=Specify via dialog  OutDataType=fixdt('single')  OutScaling=[]  DoSatur=off
  Mux : Mux  Inputs=2
  Sum : Sum  Inputs=|-+
  PercOut : Outport
  wires:
  InputBus/1 -> Bus Selector/1
  Bus Selector/3 -> Mux/2, Sum/2  "<MaxDischargeTemp>"
  Sum/1 -> Mux/1
  Bus Selector/2 -> Sum/1  "<CellTempTaper>"
  Constant/1 -> Lookup Table Dynamic/3
  Mux/1 -> Lookup Table Dynamic/2
  Bus Selector/1 -> Lookup Table Dynamic/1  "<HighCellTemp>"
  Lookup Table Dynamic/1 -> PercOut/1

== system GTA_PCMFirmware/Function/2 Control Loop/Safety/Current Limit/TorqueLimit/Low Cell Temp ==
  InputBus : Inport
  Bus Selector1 : BusSelector  OutputSignals=Input Bus.CANin.BMS.csCellTemps.LowCellTemp,Input Bus.Limits.BattLimits.MinDischargeTemp,Input Bus.SysParams.CellTempTaper
  Constant : Constant  Value=[0 100]  OutDataTypeStr=single
  Lookup Table Dynamic : simulink/Lookup Tables/Lookup Table Dynamic  LookUpMeth=Interpolation-Use End Values  OutDataTypeStr=fixdt('single')  OutputDataTypeScalingMode=Specify via dialog  OutDataType=fixdt('single')  OutScaling=[]  DoSatur=off
  Mux : Mux  Inputs=2
  Sum : Sum  Inputs=++|
  PercOut : Outport
  wires:
  InputBus/1 -> Bus Selector1/1
  Constant/1 -> Lookup Table Dynamic/3
  Mux/1 -> Lookup Table Dynamic/2
  Bus Selector1/1 -> Lookup Table Dynamic/1  "<LowCellTemp>"
  Bus Selector1/2 -> Mux/1, Sum/1  "<MinDischargeTemp>"
  Sum/1 -> Mux/2
  Bus Selector1/3 -> Sum/2  "<CellTempTaper>"
  Lookup Table Dynamic/1 -> PercOut/1

== system GTA_PCMFirmware/Function/2 Control Loop/Safety/Current Limit/TorqueLimit/Pack Voltage Limiter ==
  InputBus : Inport
  Bus Selector : BusSelector  OutputSignals=Voltage level.AvgVoltage,Input Bus.Limits.BattLimits.MinPackVoltage,Input Bus.SysParams.PackVoltageTaper
  Constant : Constant  Value=[0 100]  OutDataTypeStr=single
  Lookup Table Dynamic : simulink/Lookup Tables/Lookup Table Dynamic  LookUpMeth=Interpolation-Use End Values  OutDataTypeStr=fixdt('single')  OutputDataTypeScalingMode=Specify via dialog  OutDataType=fixdt('single')  OutScaling=[]  DoSatur=off
  Mux : Mux  Inputs=2
  Sum : Sum  Inputs=++|
  PercOut : Outport
  wires:
  InputBus/1 -> Bus Selector/1
  Bus Selector/1 -> Lookup Table Dynamic/1  "<AvgVoltage>"
  Bus Selector/2 -> Sum/1, Mux/1  "<MinPackVoltage>"
  Bus Selector/3 -> Sum/2  "<PackVoltageTaper>"
  Sum/1 -> Mux/2
  Mux/1 -> Lookup Table Dynamic/2
  Constant/1 -> Lookup Table Dynamic/3
  Lookup Table Dynamic/1 -> PercOut/1

== system GTA_PCMFirmware/Function/2 Control Loop/Safety/Current Limit/TorqueLimit/SOC Limiter ==
  InputBus : Inport
  Bus Selector : BusSelector  OutputSignals=Input Bus.CANin.BMS.csInfo.UserSOC,Input Bus.SysParams.LowSOCcurrLimit
  Constant : Constant  Value=100  OutDataTypeStr=single
  Constant1 : Constant  Value=[0 1]  OutDataTypeStr=single
  Lookup Table Dynamic : simulink/Lookup Tables/Lookup Table Dynamic  LookUpMeth=Interpolation-Use End Values  OutDataTypeStr=fixdt('single')  OutputDataTypeScalingMode=Specify via dialog  OutDataType=fixdt('single')  OutScaling=[]  DoSatur=off
  Mux : Mux  Inputs=2
  PercOut : Outport
  wires:
  InputBus/1 -> Bus Selector/1
  Bus Selector/1 -> Lookup Table Dynamic/1  "<UserSOC>"
  Bus Selector/2 -> Mux/1  "<LowSOCcurrLimit>"
  Constant/1 -> Mux/2
  Mux/1 -> Lookup Table Dynamic/3
  Constant1/1 -> Lookup Table Dynamic/2
  Lookup Table Dynamic/1 -> PercOut/1

== system GTA_PCMFirmware/Function/2 Control Loop/Safety/Current Limit/TorqueLimit/Speed Limiter ==
  InputBus : Inport
  % : Constant  Value=[-100 0 100 100 0 -100]  OutDataTypeStr=single
  Add1 : Sum  Inputs=|-+
  Add2 : Sum  Inputs=++|
  Add3 : Sum  Inputs=|-+
  Add4 : Sum  Inputs=++|
  Bus Selector : BusSelector  OutputSignals=Input Bus.CANin.Motor Controller.KinVoltSpeed.SpeedLPF,Input Bus.SysParams.SpeedTaper,Input Bus.SysParams.RevSpeedLimit,Input Bus.CANin.BMS.csInfo.csSOC,Input Bus.SysParams.MinSOC,Input Bus.SysParams.HighSpeedLimit,Input Bus.SysParams.LowSpeedLimit
  Lookup Table Dynamic : simulink/Lookup Tables/Lookup Table Dynamic  LookUpMeth=Interpolation-Use End Values  OutDataTypeStr=fixdt('single')  OutputDataTypeScalingMode=Specify via dialog  OutDataType=fixdt('single')  OutScaling=[]  DoSatur=off
  Multiport Switch : MultiPortSwitch  DataPortOrder=Zero-based contiguous  Inputs=2  zeroidx=on
  Mux : Mux  Inputs=6
  Relational Operator1 : RelationalOperator  Operator=<=  OutDataTypeStr=boolean
  motohawk_probe1 : MotoHawk_lib/Calibration & Probing Blocks/motohawk_probe  nam='SpeedlimiterXDAT'  show_more=on  name_source=Use Parameter  read_level=1  view_as=Number  enum_struct={'Disabled', 'Enabled'}  vector_style=Wide Row  use_help_units=off  help=''  units=''  use_header_enum=off  row_header_enum={}  col_header_enum={}  use_min_max=off  min_val=-inf  max_val=inf  use_precision=off  precision=''  gain=1  offset=0  exp=1  use_mototune_group=off  mototune_group=motohawk_vardec_path(gcb)
  motohawk_probe2 : MotoHawk_lib/Calibration & Probing Blocks/motohawk_probe  nam='SpeedlimiterYDAT'  show_more=on  name_source=Use Parameter  read_level=1  view_as=Number  enum_struct={'Disabled', 'Enabled'}  vector_style=Wide Row  use_help_units=off  help=''  units=''  use_header_enum=off  row_header_enum={}  col_header_enum={}  use_min_max=off  min_val=-inf  max_val=inf  use_precision=off  precision=''  gain=1  offset=0  exp=1  use_mototune_group=off  mototune_group=motohawk_vardec_path(gcb)
  PercentOut : Outport
  wires:
  InputBus/1 -> Bus Selector/1
  Relational Operator1/1 -> Multiport Switch/1
  Bus Selector/4 -> Relational Operator1/1  "<csSOC>"
  Bus Selector/5 -> Relational Operator1/2  "<MinSOC>"
  Bus Selector/6 -> Multiport Switch/2  "<HighSpeedLimit>"
  Bus Selector/7 -> Multiport Switch/3  "<LowSpeedLimit>"
  Add1/1 -> Mux/1
  Add2/1 -> Mux/3
  Add3/1 -> Mux/4
  Add4/1 -> Mux/6
  Multiport Switch/1 -> Mux/5, Add3/2, Add4/1  "HighSpped"
  Bus Selector/3 -> Mux/2, Add2/1, Add1/2  "<RevSpeedLimit>"
  Bus Selector/2 -> Add4/2, Add3/1, Add2/2, Add1/1  "<SpeedTaper>"
  Mux/1 -> motohawk_probe1/1, Lookup Table Dynamic/2
  %/1 -> motohawk_probe2/1, Lookup Table Dynamic/3
  Bus Selector/1 -> Lookup Table Dynamic/1  "<SpeedLPF>"
  Lookup Table Dynamic/1 -> PercentOut/1

== system GTA_PCMFirmware/Function/2 Control Loop/Safety/Faults/BatteryFault/Filter ==
  In1 : Inport
  Delay : Delay  DelayLength=200
  Logical Operator : Logic  AllPortsSameDT=off  OutDataTypeStr=boolean
  Out1 : Outport
  wires:
  Delay/1 -> Logical Operator/2
  In1/1 -> Delay/1, Logical Operator/1
  Logical Operator/1 -> Out1/1
